simulink model "sscoutputfeedback"  (R2016a)
settings: Solver=VariableStepAuto  StartTime=0.0  StopTime=10.0  RelTol=1e-3
values from neighbouring files (symbols this model uses):
  r = 3    [parameters.m]
  sigma = 2    [configuration.m]    (also in parameters.m = 1)
  tau = 1    [configuration.m]    (also in parameters.m = 0.1)
settings Model: Creator=Gabriel-Lenovo  LastModifiedBy=Gabriel-Lenovo

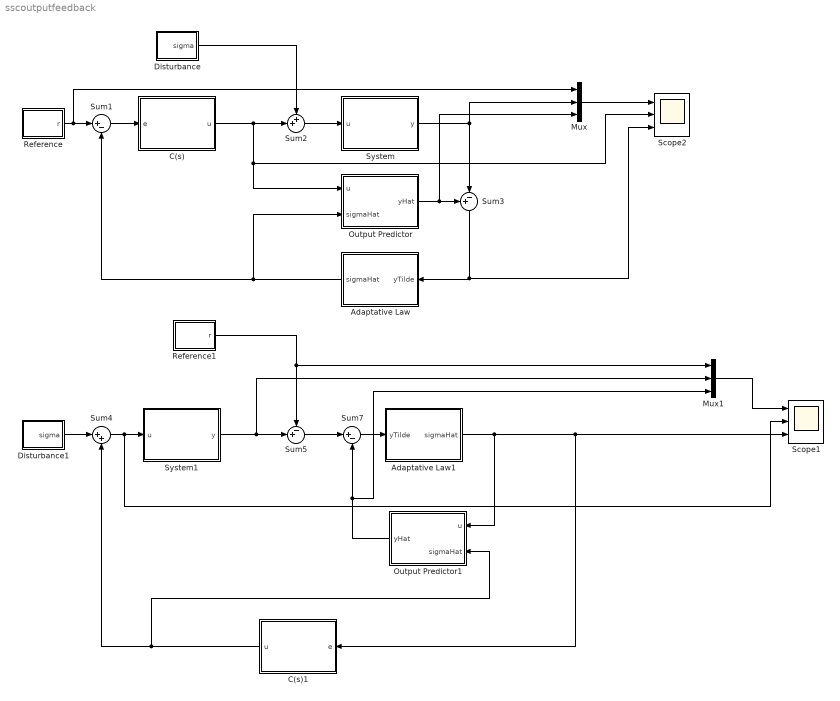
== system sscoutputfeedback ==
  Adaptative Law : Subsystem
  Adaptative Law1 : Subsystem
  C(s) : Subsystem
  C(s)1 : Subsystem
  Disturbance : Subsystem
  Disturbance1 : Subsystem
  Mux : Mux  Inputs=3
  Mux1 : Mux  Inputs=3
  Output Predictor : Subsystem
  Output Predictor1 : Subsystem
  Reference : Subsystem
  Reference1 : Subsystem
  Scope1 : Scope  NumInputPorts=3
  Scope2 : Scope  NumInputPorts=3
  Sum1 : Sum  Inputs=|+-
  Sum2 : Sum  Inputs=++|
  Sum3 : Sum  Inputs=+-|
  Sum4 : Sum  Inputs=|++
  Sum5 : Sum  Inputs=-+|
  Sum7 : Sum  Inputs=|+-
  System : Subsystem
  System1 : Subsystem
  wires:
  Sum1/1 -> C(s)/1(e)
  Adaptative Law/1(sigmaHat) -> Sum1/2, Output Predictor/2(sigmaHat)
  Reference/1(r) -> Mux/1, Sum1/1
  Output Predictor/1(yHat) -> Mux/3, Sum3/1
  System/1(y) -> Mux/2, Sum3/2
  Disturbance/1(sigma) -> Sum2/1
  C(s)/1(u) -> Output Predictor/1("u "), Scope2/2, Sum2/2
  Sum2/1 -> System/1(u)
  Mux/1 -> Scope2/1
  Sum3/1 -> Scope2/3, Adaptative Law/1(yTilde)
  Sum4/1 -> Scope1/2, System1/1(u)
  Disturbance1/1(sigma) -> Sum4/1
  System1/1(y) -> Mux1/2, Sum5/2
  Sum5/1 -> Sum7/1
  Mux1/1 -> Scope1/1
  Sum7/1 -> Adaptative Law1/1(yTilde)
  Adaptative Law1/1(sigmaHat) -> Output Predictor1/1("u "), C(s)1/1(e), Scope1/3
  C(s)1/1(u) -> Output Predictor1/2(sigmaHat), Sum4/2
  Output Predictor1/1(yHat) -> Mux1/3, Sum7/2
  Reference1/1(r) -> Sum5/1, Mux1/1

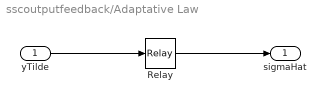
== system sscoutputfeedback/Adaptative Law ==
  yTilde : Inport
  Relay : Relay  OffOutputValue=-1
  sigmaHat : Outport
  wires:
  yTilde/1 -> Relay/1
  Relay/1 -> sigmaHat/1

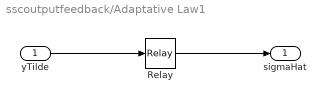
== system sscoutputfeedback/Adaptative Law1 ==
  yTilde : Inport
  Relay : Relay
  sigmaHat : Outport
  wires:
  yTilde/1 -> Relay/1
  Relay/1 -> sigmaHat/1

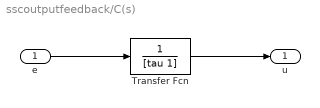
== system sscoutputfeedback/C(s) ==
  e : Inport
  Transfer Fcn : TransferFcn  Denominator=[tau 1]
  u : Outport
  wires:
  e/1 -> Transfer Fcn/1
  Transfer Fcn/1 -> u/1

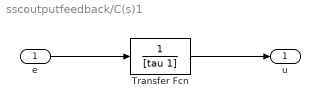
== system sscoutputfeedback/C(s)1 ==
  e : Inport
  Transfer Fcn : TransferFcn  Denominator=[tau 1]
  u : Outport
  wires:
  e/1 -> Transfer Fcn/1
  Transfer Fcn/1 -> u/1

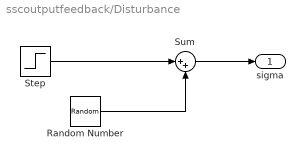
== system sscoutputfeedback/Disturbance ==
  Random Number : RandomNumber  Variance=0
  Step : Step  Time=10  After=sigma*2  SampleTime=0
  Sum : Sum  Inputs=|++
  sigma : Outport
  wires:
  Step/1 -> Sum/1
  Random Number/1 -> Sum/2
  Sum/1 -> sigma/1

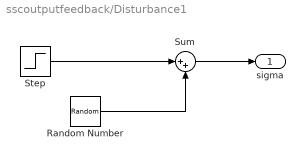
== system sscoutputfeedback/Disturbance1 ==
  Random Number : RandomNumber  Variance=0
  Step : Step  Time=10  After=sigma*2  SampleTime=0
  Sum : Sum  Inputs=|++
  sigma : Outport
  wires:
  Step/1 -> Sum/1
  Random Number/1 -> Sum/2
  Sum/1 -> sigma/1

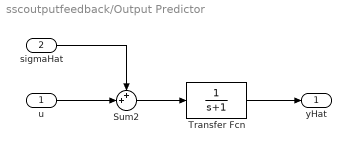
== system sscoutputfeedback/Output Predictor ==
  "u " : Inport
  sigmaHat : Inport  Port=2
  Sum2 : Sum  Inputs=++|
  Transfer Fcn : TransferFcn  Denominator=[1 1]
  yHat : Outport
  wires:
  Transfer Fcn/1 -> yHat/1
  "u "/1 -> Sum2/2
  sigmaHat/1 -> Sum2/1
  Sum2/1 -> Transfer Fcn/1

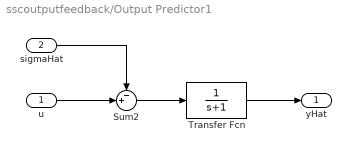
== system sscoutputfeedback/Output Predictor1 ==
  "u " : Inport
  sigmaHat : Inport  Port=2
  Sum2 : Sum  Inputs=-+|
  Transfer Fcn : TransferFcn  Denominator=[1 1]
  yHat : Outport
  wires:
  Transfer Fcn/1 -> yHat/1
  "u "/1 -> Sum2/2
  sigmaHat/1 -> Sum2/1
  Sum2/1 -> Transfer Fcn/1

== system sscoutputfeedback/Reference ==
  Step : Step  After=r  SampleTime=0
  r : Outport
  wires:
  Step/1 -> r/1

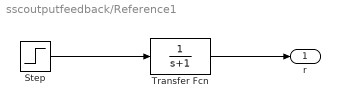
== system sscoutputfeedback/Reference1 ==
  Step : Step  After=r  SampleTime=0
  Transfer Fcn : TransferFcn  Denominator=[1 1]
  r : Outport
  wires:
  Step/1 -> Transfer Fcn/1
  Transfer Fcn/1 -> r/1

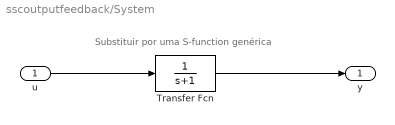
== system sscoutputfeedback/System ==
  note: Substituir por uma S-function genérica
  u : Inport
  Transfer Fcn : TransferFcn  Denominator=[1 1]
  y : Outport
  wires:
  u/1 -> Transfer Fcn/1
  Transfer Fcn/1 -> y/1

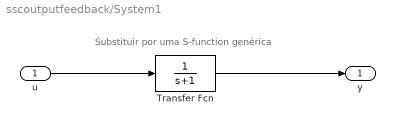
== system sscoutputfeedback/System1 ==
  note: Substituir por uma S-function genérica
  u : Inport
  Transfer Fcn : TransferFcn  Denominator=[1 1]
  y : Outport
  wires:
  u/1 -> Transfer Fcn/1
  Transfer Fcn/1 -> y/1
